simulink library "THLlib"  (R2017a)
settings: Solver=ode45  StartTime=0.0  StopTime=10.0  RelTol=1e-3  EnableMultiTasking=on
PostLoadFcn:
  | setsysloc(bdroot)
StartFcn:
  | open_system('MinSegLibrary','force')
libraries: arduinolib x6
settings Model: Creator=hurstj  LastModifiedBy=student
settings DataIOCC: LimitDataPoints=on  SaveFormat=Array  SignalLoggingSaveFormat=ModelDataLogs
settings OptimizationCC: LifeSpan=inf
settings DebuggingCC: UnderspecifiedInitializationDetection=Classic  MergeDetectMultiDrivingBlocksExec=none  SolverPrmCheckMsg=warning  MultiTaskDSMMsg=warning  MultiTaskCondExecSysMsg=none  StateNameClashWarn=warning  StrictBusMsg=None  SFUnexpectedBacktrackingDiag=warning  SFNoUnconditionalDefaultTransitionDiag=warning  SFExecutionAtInitializationDiag=none
settings HardwareCC: ProdBitPerPointer=32  ProdBitPerSizeT=32  ProdBitPerPtrDiffT=32  ProdLargestAtomicFloat=None  ProdIntDivRoundTo=Undefined  ProdEndianess=Unspecified  ProdWordSize=32  ProdHWDeviceType=32-bit Generic
settings ModelReferenceCC: PropagateSignalLabelsOutOfModel=off
settings GRTTargetCC: TargetLangStandard=C89/C90 (ANSI)  GeneratePreprocessorConditionals=Disable all
settings ConfigComp: CovMetricSettings=dw  CovHtmlReporting=on  CovSaveCumulativeToWorkspaceVar=on  CovSaveSingleToWorkspaceVar=on  CovExternalEMLEnable=off

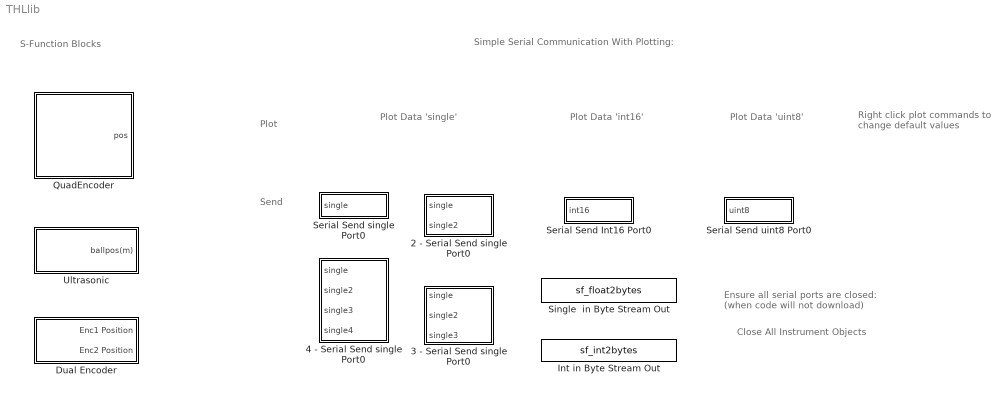
== system THLlib ==
  note: Right click
      |  plot commands
      | to change
      | default values
  note: Ensure all serial ports are closed:
      | (when code will not download)
  note: Plot
  note: Send
  note: Plot Data
      | 'int16'
  note: Plot Data
      | 'single'
  note: Plot Data
      | 'uint8'
  note: Simple Serial Communication
      | With Plotting:
  note: Close All
      | Instrument Objects
  note: S-Function Blocks
  2 - Serial Send single Port0 : Subsystem
  3 - Serial Send single Port0 : Subsystem  AncestorBlock="CSLlib/2 - Serial Send  single Port0"
  4 - Serial Send single Port0 : Subsystem  AncestorBlock="CSLlib/3 - Serial Send  single Port0"
  Dual Encoder : Subsystem
  Int in Byte Stream Out : S-Function  InitFcn=try, set_param(gcb,'FunctionName','sf_int2bytes'), end  FunctionName=sf_int2bytes  SFunctionModules=sf_int2bytes_wrapper  SFunctionDeploymentMode=off  EnableBusSupport=off  mask(S-Function Builder){}
      mask init:
      | val = [[.9  0.75 0.75 1 1 .9 .9 1]',[1 1 0.75 0.75 .9 .9 1 .9]'];try , sys = get_param(gcb,'SfunBuilderFcnName');if isempty(sys), sys = get_param(gcb,'FunctionName'); end,catch, sys = get_param(gcb,'FunctionName'); end
      settings: CopyFcn=set_param(gcb,'LinkStatus','none')  PreSaveFcn=try, set_param(gcb,'FunctionName','sf_int2bytes'), end  OpenFcn=sfunctionwizard(gcbh)
      mask Display: plot(val(:,1),val(:,2)),disp(sys), port_label('input',1,'int_in'), port_label('output',1,'bout')
  QuadEncoder : Subsystem
  Serial Send Int16 Port0 : Subsystem
  Serial Send single Port0 : Subsystem
  Serial Send uint8 Port0 : Subsystem
  Single  in Byte Stream Out : S-Function  InitFcn=try, set_param(gcb,'FunctionName','sf_float2bytes'), end  FunctionName=sf_float2bytes  SFunctionModules=sf_float2bytes_wrapper  SFunctionDeploymentMode=off  EnableBusSupport=off  mask(S-Function Builder){}
      mask init: same as THLlib/Int in Byte Stream Out
      settings: CopyFcn=set_param(gcb,'LinkStatus','none')  PreSaveFcn=try, set_param(gcb,'FunctionName','sf_float2bytes'), end  OpenFcn=sfunctionwizard(gcbh)
      mask Display: plot(val(:,1),val(:,2)),disp(sys), port_label('input',1,'fin'), port_label('output',1,'bout')
  Ultrasonic : Subsystem

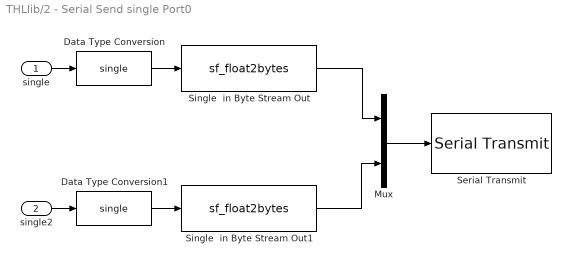
== system THLlib/2 - Serial Send single Port0 ==
  single : Inport
  single2 : Inport  Port=2
  Data Type Conversion : DataTypeConversion  OutDataTypeStr=single
  Data Type Conversion1 : DataTypeConversion  OutDataTypeStr=single
  Mux : Mux  Inputs=2
  Serial Transmit : arduinolib/Serial Transmit  portNumber=0
      settings: SourceProductName=Simulink Support Package for Arduino Hardware
  Single  in Byte Stream Out : S-Function  InitFcn=try, set_param(gcb,'FunctionName','sf_float2bytes'), end  FunctionName=sf_float2bytes  SFunctionModules=sf_float2bytes_wrapper  SFunctionDeploymentMode=off  EnableBusSupport=off  mask(S-Function Builder){}
      mask init: same as THLlib/Int in Byte Stream Out
      settings: CopyFcn=set_param(gcb,'LinkStatus','none')  PreSaveFcn=try, set_param(gcb,'FunctionName','sf_float2bytes'), end  OpenFcn=sfunctionwizard(gcbh)
      mask Display: plot(val(:,1),val(:,2)),disp(sys), port_label('input',1,'fin'), port_label('output',1,'bout')
  Single  in Byte Stream Out1 : S-Function  InitFcn=try, set_param(gcb,'FunctionName','sf_float2bytes'), end  FunctionName=sf_float2bytes  SFunctionModules=sf_float2bytes_wrapper  SFunctionDeploymentMode=off  EnableBusSupport=off  mask(S-Function Builder){}
      mask init: same as THLlib/Int in Byte Stream Out
      settings: CopyFcn=set_param(gcb,'LinkStatus','none')  PreSaveFcn=try, set_param(gcb,'FunctionName','sf_float2bytes'), end  OpenFcn=sfunctionwizard(gcbh)
      mask Display: plot(val(:,1),val(:,2)),disp(sys), port_label('input',1,'fin'), port_label('output',1,'bout')
  wires:
  Mux/1 -> Serial Transmit/1
  Single  in Byte Stream Out/1 -> Mux/1
  Single  in Byte Stream Out1/1 -> Mux/2
  Data Type Conversion1/1 -> Single  in Byte Stream Out1/1
  single2/1 -> Data Type Conversion1/1
  Data Type Conversion/1 -> Single  in Byte Stream Out/1
  single/1 -> Data Type Conversion/1

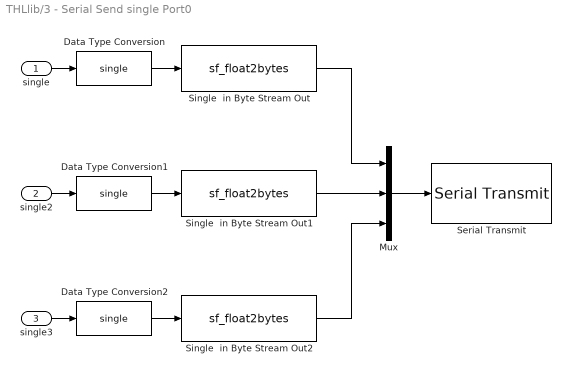
== system THLlib/3 - Serial Send single Port0 ==
  single : Inport
  single2 : Inport  Port=2
  single3 : Inport  Port=3
  Data Type Conversion : DataTypeConversion  OutDataTypeStr=single
  Data Type Conversion1 : DataTypeConversion  OutDataTypeStr=single
  Data Type Conversion2 : DataTypeConversion  OutDataTypeStr=single
  Mux : Mux  Inputs=3
  Serial Transmit : arduinolib/Serial Transmit  portNumber=0
      settings: SourceProductName=Simulink Support Package for Arduino Hardware
  Single  in Byte Stream Out : S-Function  InitFcn=try, set_param(gcb,'FunctionName','sf_float2bytes'), end  FunctionName=sf_float2bytes  SFunctionModules=sf_float2bytes_wrapper  SFunctionDeploymentMode=off  EnableBusSupport=off  mask(S-Function Builder){}
      mask init: same as THLlib/Int in Byte Stream Out
      settings: CopyFcn=set_param(gcb,'LinkStatus','none')  PreSaveFcn=try, set_param(gcb,'FunctionName','sf_float2bytes'), end  OpenFcn=sfunctionwizard(gcbh)
      mask Display: plot(val(:,1),val(:,2)),disp(sys), port_label('input',1,'fin'), port_label('output',1,'bout')
  Single  in Byte Stream Out1 : S-Function  InitFcn=try, set_param(gcb,'FunctionName','sf_float2bytes'), end  FunctionName=sf_float2bytes  SFunctionModules=sf_float2bytes_wrapper  SFunctionDeploymentMode=off  EnableBusSupport=off  mask(S-Function Builder){}
      mask init: same as THLlib/Int in Byte Stream Out
      settings: CopyFcn=set_param(gcb,'LinkStatus','none')  PreSaveFcn=try, set_param(gcb,'FunctionName','sf_float2bytes'), end  OpenFcn=sfunctionwizard(gcbh)
      mask Display: plot(val(:,1),val(:,2)),disp(sys), port_label('input',1,'fin'), port_label('output',1,'bout')
  Single  in Byte Stream Out2 : S-Function  InitFcn=try, set_param(gcb,'FunctionName','sf_float2bytes'), end  FunctionName=sf_float2bytes  SFunctionModules=sf_float2bytes_wrapper  SFunctionDeploymentMode=off  EnableBusSupport=off  mask(S-Function Builder){}
      mask init: same as THLlib/Int in Byte Stream Out
      settings: CopyFcn=set_param(gcb,'LinkStatus','none')  PreSaveFcn=try, set_param(gcb,'FunctionName','sf_float2bytes'), end  OpenFcn=sfunctionwizard(gcbh)
      mask Display: plot(val(:,1),val(:,2)),disp(sys), port_label('input',1,'fin'), port_label('output',1,'bout')
  wires:
  single/1 -> Data Type Conversion/1
  Data Type Conversion/1 -> Single  in Byte Stream Out/1
  single2/1 -> Data Type Conversion1/1
  Data Type Conversion1/1 -> Single  in Byte Stream Out1/1
  Single  in Byte Stream Out1/1 -> Mux/2
  Single  in Byte Stream Out/1 -> Mux/1
  Mux/1 -> Serial Transmit/1
  single3/1 -> Data Type Conversion2/1
  Data Type Conversion2/1 -> Single  in Byte Stream Out2/1
  Single  in Byte Stream Out2/1 -> Mux/3

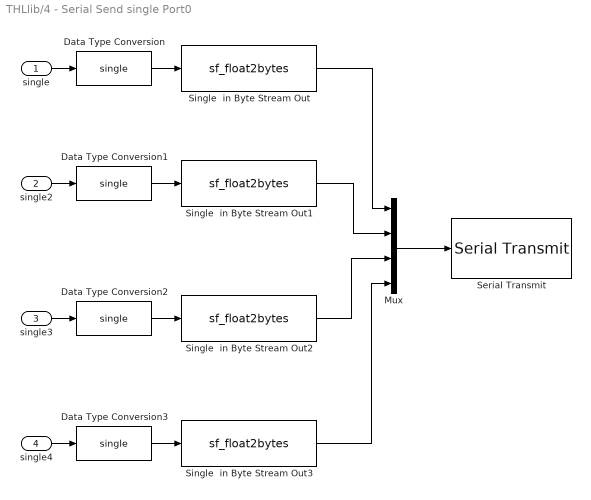
== system THLlib/4 - Serial Send single Port0 ==
  single : Inport
  single2 : Inport  Port=2
  single3 : Inport  Port=3
  single4 : Inport  Port=4
  Data Type Conversion{,1..3} (4 alike) : DataTypeConversion  OutDataTypeStr=single
  Mux : Mux
  Serial Transmit : arduinolib/Serial Transmit  portNumber=0
      settings: SourceProductName=Simulink Support Package for Arduino Hardware
  Single  in Byte Stream Out : S-Function  InitFcn=try, set_param(gcb,'FunctionName','sf_float2bytes'), end  FunctionName=sf_float2bytes  SFunctionModules=sf_float2bytes_wrapper  SFunctionDeploymentMode=off  EnableBusSupport=off  mask(S-Function Builder){}
      mask init: same as THLlib/Int in Byte Stream Out
      settings: CopyFcn=set_param(gcb,'LinkStatus','none')  PreSaveFcn=try, set_param(gcb,'FunctionName','sf_float2bytes'), end  OpenFcn=sfunctionwizard(gcbh)
      mask Display: plot(val(:,1),val(:,2)),disp(sys), port_label('input',1,'fin'), port_label('output',1,'bout')
  Single  in Byte Stream Out1 : S-Function  InitFcn=try, set_param(gcb,'FunctionName','sf_float2bytes'), end  FunctionName=sf_float2bytes  SFunctionModules=sf_float2bytes_wrapper  SFunctionDeploymentMode=off  EnableBusSupport=off  mask(S-Function Builder){}
      mask init: same as THLlib/Int in Byte Stream Out
      settings: CopyFcn=set_param(gcb,'LinkStatus','none')  PreSaveFcn=try, set_param(gcb,'FunctionName','sf_float2bytes'), end  OpenFcn=sfunctionwizard(gcbh)
      mask Display: plot(val(:,1),val(:,2)),disp(sys), port_label('input',1,'fin'), port_label('output',1,'bout')
  Single  in Byte Stream Out2 : S-Function  InitFcn=try, set_param(gcb,'FunctionName','sf_float2bytes'), end  FunctionName=sf_float2bytes  SFunctionModules=sf_float2bytes_wrapper  SFunctionDeploymentMode=off  EnableBusSupport=off  mask(S-Function Builder){}
      mask init: same as THLlib/Int in Byte Stream Out
      settings: CopyFcn=set_param(gcb,'LinkStatus','none')  PreSaveFcn=try, set_param(gcb,'FunctionName','sf_float2bytes'), end  OpenFcn=sfunctionwizard(gcbh)
      mask Display: plot(val(:,1),val(:,2)),disp(sys), port_label('input',1,'fin'), port_label('output',1,'bout')
  Single  in Byte Stream Out3 : S-Function  InitFcn=try, set_param(gcb,'FunctionName','sf_float2bytes'), end  FunctionName=sf_float2bytes  SFunctionModules=sf_float2bytes_wrapper  SFunctionDeploymentMode=off  EnableBusSupport=off  mask(S-Function Builder){}
      mask init: same as THLlib/Int in Byte Stream Out
      settings: CopyFcn=set_param(gcb,'LinkStatus','none')  PreSaveFcn=try, set_param(gcb,'FunctionName','sf_float2bytes'), end  OpenFcn=sfunctionwizard(gcbh)
      mask Display: plot(val(:,1),val(:,2)),disp(sys), port_label('input',1,'fin'), port_label('output',1,'bout')
  wires:
  Single  in Byte Stream Out2/1 -> Mux/3
  Data Type Conversion2/1 -> Single  in Byte Stream Out2/1
  single3/1 -> Data Type Conversion2/1
  Mux/1 -> Serial Transmit/1
  Single  in Byte Stream Out/1 -> Mux/1
  Single  in Byte Stream Out1/1 -> Mux/2
  Data Type Conversion1/1 -> Single  in Byte Stream Out1/1
  single2/1 -> Data Type Conversion1/1
  Data Type Conversion/1 -> Single  in Byte Stream Out/1
  single/1 -> Data Type Conversion/1
  Data Type Conversion3/1 -> Single  in Byte Stream Out3/1
  single4/1 -> Data Type Conversion3/1
  Single  in Byte Stream Out3/1 -> Mux/4

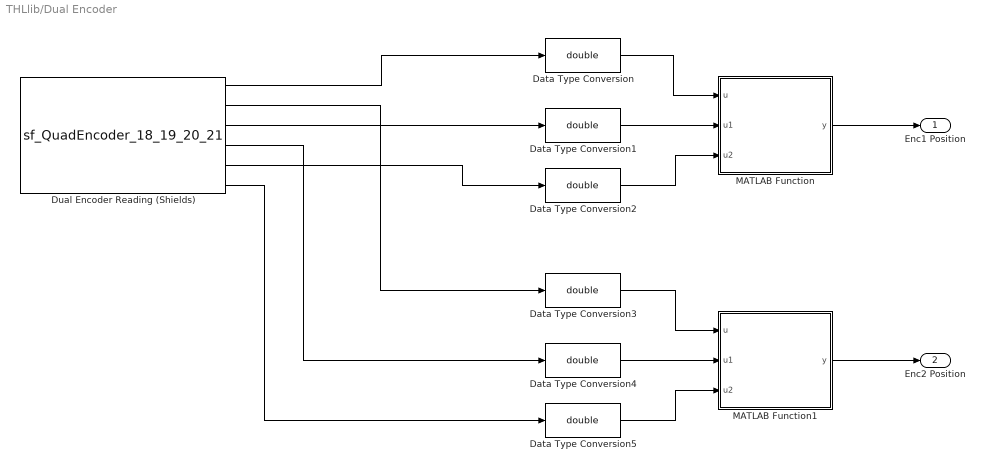
== system THLlib/Dual Encoder ==
  Data Type Conversion{,1..5} (6 alike) : DataTypeConversion  OutDataTypeStr=double
  Dual Encoder Reading (Shields) : S-Function  InitFcn=try, set_param(gcb,'FunctionName','sf_QuadEncoder_18_19_20_21'), end  FunctionName=sf_QuadEncoder_18_19_20_21  Parameters=uint8([0 1]),uint8([18 20]),uint8([19 21])  SFunctionModules=sf_QuadEncoder_18_19_20_21_wrapper  SFunctionDeploymentMode=off  EnableBusSupport=off  mask(S-Function Builder){}
      mask init: same as THLlib/Int in Byte Stream Out
      settings: CopyFcn=set_param(gcbh,'LinkStatus','none')  PreSaveFcn=try, set_param(gcb,'FunctionName','sf_QuadEncoder_18_19_20_21'), end  OpenFcn=sfunctionwizard(gcbh)
      mask Display: plot(val(:,1),val(:,2)),disp(sys), port_label('output',1,'pos1'), port_label('output',2,'pos2'), port_label('output',3,'OF1'), port_label('output',4,'OF2'), port_label('output',5,'UF1'), port_label('output',6,'UF2')
  MATLAB Function : Subsystem  TreatAsAtomicUnit=on
  MATLAB Function1 : Subsystem  TreatAsAtomicUnit=on
  Enc1 Position : Outport
  Enc2 Position : Outport  Port=2
  wires:
  MATLAB Function1/1(y) -> Enc2 Position/1
  MATLAB Function/1(y) -> Enc1 Position/1
  Data Type Conversion5/1 -> MATLAB Function1/3(u2)
  Data Type Conversion4/1 -> MATLAB Function1/2(u1)
  Data Type Conversion3/1 -> MATLAB Function1/1(u)
  Data Type Conversion2/1 -> MATLAB Function/3(u2)
  Data Type Conversion1/1 -> MATLAB Function/2(u1)
  Data Type Conversion/1 -> MATLAB Function/1(u)
  Dual Encoder Reading (Shields)/6 -> Data Type Conversion5/1
  Dual Encoder Reading (Shields)/5 -> Data Type Conversion2/1
  Dual Encoder Reading (Shields)/4 -> Data Type Conversion4/1
  Dual Encoder Reading (Shields)/3 -> Data Type Conversion1/1
  Dual Encoder Reading (Shields)/2 -> Data Type Conversion3/1
  Dual Encoder Reading (Shields)/1 -> Data Type Conversion/1

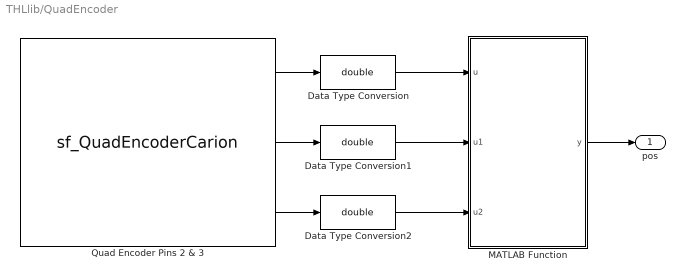
== system THLlib/QuadEncoder ==
  Data Type Conversion : DataTypeConversion  OutDataTypeStr=double
  Data Type Conversion1 : DataTypeConversion  OutDataTypeStr=double
  Data Type Conversion2 : DataTypeConversion  OutDataTypeStr=double
  MATLAB Function : MATLAB Function  TreatAsAtomicUnit=on
  Quad Encoder Pins 2 & 3 : S-Function  InitFcn=try, set_param(gcb,'FunctionName','sf_QuadEncoderCarion'), end  FunctionName=sf_QuadEncoderCarion  Parameters=uint8(0),uint8(2),uint8(3)  SFunctionModules=sf_QuadEncoderCarion_wrapper  SFunctionDeploymentMode=off  EnableBusSupport=off  mask(S-Function Builder){}
      mask init: same as THLlib/Int in Byte Stream Out
      settings: CopyFcn=set_param(gcbh,'LinkStatus','none')  PreSaveFcn=try, set_param(gcb,'FunctionName','sf_QuadEncoderCarion'), end  OpenFcn=sfunctionwizard(gcbh)
      mask Display: plot(val(:,1),val(:,2)),disp(sys), port_label('output',1,'pos'), port_label('output',2,'overflow'), port_label('output',3,'underflow')
  pos : Outport
  wires:
  Quad Encoder Pins 2 & 3/3 -> Data Type Conversion2/1
  Quad Encoder Pins 2 & 3/2 -> Data Type Conversion1/1
  MATLAB Function/1(y) -> pos/1
  Quad Encoder Pins 2 & 3/1 -> Data Type Conversion/1
  Data Type Conversion2/1 -> MATLAB Function/3(u2)
  Data Type Conversion1/1 -> MATLAB Function/2(u1)
  Data Type Conversion/1 -> MATLAB Function/1(u)

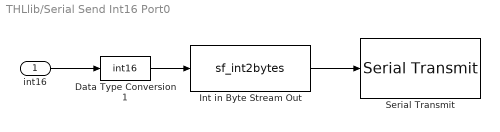
== system THLlib/Serial Send Int16 Port0 ==
  int16 : Inport
  Data Type Conversion1 : DataTypeConversion  OutDataTypeStr=int16
  Int in Byte Stream Out : S-Function  InitFcn=try, set_param(gcb,'FunctionName','sf_int2bytes'), end  FunctionName=sf_int2bytes  SFunctionModules=sf_int2bytes_wrapper  SFunctionDeploymentMode=off  EnableBusSupport=off  mask(S-Function Builder){}
      mask init: same as THLlib/Int in Byte Stream Out
      settings: CopyFcn=set_param(gcb,'LinkStatus','none')  PreSaveFcn=try, set_param(gcb,'FunctionName','sf_int2bytes'), end  OpenFcn=sfunctionwizard(gcbh)
      mask Display: plot(val(:,1),val(:,2)),disp(sys), port_label('input',1,'int_in'), port_label('output',1,'bout')
  Serial Transmit : arduinolib/Serial Transmit  portNumber=0
      settings: SourceProductName=Simulink Support Package for Arduino Hardware
  wires:
  Data Type Conversion1/1 -> Int in Byte Stream Out/1
  int16/1 -> Data Type Conversion1/1
  Int in Byte Stream Out/1 -> Serial Transmit/1

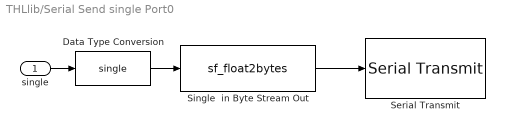
== system THLlib/Serial Send single Port0 ==
  single : Inport
  Data Type Conversion : DataTypeConversion  OutDataTypeStr=single
  Serial Transmit : arduinolib/Serial Transmit  portNumber=0
      settings: SourceProductName=Simulink Support Package for Arduino Hardware
  Single  in Byte Stream Out : S-Function  InitFcn=try, set_param(gcb,'FunctionName','sf_float2bytes'), end  FunctionName=sf_float2bytes  SFunctionModules=sf_float2bytes_wrapper  SFunctionDeploymentMode=off  EnableBusSupport=off  mask(S-Function Builder){}
      mask init: same as THLlib/Int in Byte Stream Out
      settings: CopyFcn=set_param(gcb,'LinkStatus','none')  PreSaveFcn=try, set_param(gcb,'FunctionName','sf_float2bytes'), end  OpenFcn=sfunctionwizard(gcbh)
      mask Display: plot(val(:,1),val(:,2)),disp(sys), port_label('input',1,'fin'), port_label('output',1,'bout')
  wires:
  Single  in Byte Stream Out/1 -> Serial Transmit/1
  Data Type Conversion/1 -> Single  in Byte Stream Out/1
  single/1 -> Data Type Conversion/1

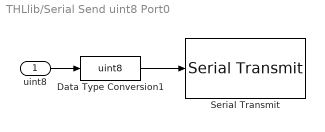
== system THLlib/Serial Send uint8 Port0 ==
  uint8 : Inport
  Data Type Conversion1 : DataTypeConversion  OutDataTypeStr=uint8
  Serial Transmit : arduinolib/Serial Transmit  portNumber=0
      settings: SourceProductName=Simulink Support Package for Arduino Hardware
  wires:
  uint8/1 -> Data Type Conversion1/1
  Data Type Conversion1/1 -> Serial Transmit/1

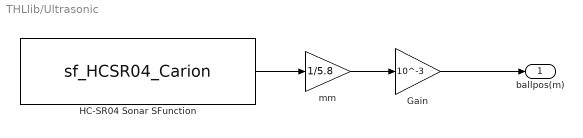
== system THLlib/Ultrasonic ==
  Gain : Gain  Gain=10^-3
  HC-SR04 Sonar SFunction : S-Function  InitFcn=try, set_param(gcb,'FunctionName','sf_HCSR04_Carion'), end  FunctionName=sf_HCSR04_Carion  SFunctionModules=sf_HCSR04_Carion_wrapper  SFunctionDeploymentMode=off  EnableBusSupport=off  mask(S-Function Builder){}
      mask help: Simulink:masks:SFunctionBuilder_MD
      mask init: same as THLlib/Int in Byte Stream Out
      settings: CopyFcn=set_param(gcbh,'LinkStatus','none')  PreSaveFcn=try, set_param(gcb,'FunctionName','sf_HCSR04_Carion'), end  OpenFcn=sfunctionwizard(gcbh)
      mask Display: plot(val(:,1),val(:,2)),disp(sys), port_label('output',1,'distance_us')
  mm : Gain  Gain=1/5.8
  ballpos(m) : Outport
  wires:
  Gain/1 -> ballpos(m)/1
  mm/1 -> Gain/1
  HC-SR04 Sonar SFunction/1 -> mm/1

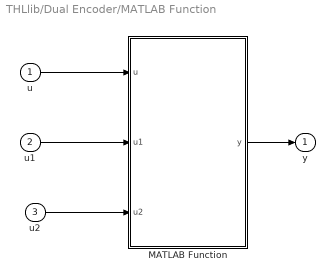
== system THLlib/Dual Encoder/MATLAB Function ==
  u : Inport
  u1 : Inport  Port=2
  u2 : Inport  Port=3
  MATLAB Function : MATLAB Function  TreatAsAtomicUnit=on
  y : Outport
  wires:
  MATLAB Function/1(y) -> y/1
  u1/1 -> MATLAB Function/2(u1)
  u2/1 -> MATLAB Function/3(u2)
  u/1 -> MATLAB Function/1(u)

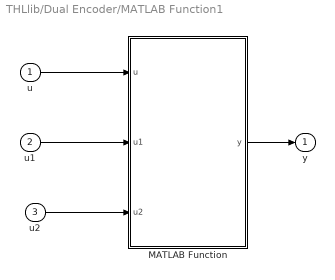
== system THLlib/Dual Encoder/MATLAB Function1 ==
  u : Inport
  u1 : Inport  Port=2
  u2 : Inport  Port=3
  MATLAB Function : MATLAB Function  TreatAsAtomicUnit=on
  y : Outport
  wires:
  MATLAB Function/1(y) -> y/1
  u1/1 -> MATLAB Function/2(u1)
  u2/1 -> MATLAB Function/3(u2)
  u/1 -> MATLAB Function/1(u)

== matlab function THLlib/QuadEncoder/MATLAB Function ==
  data: u input; y output; u1 input; u2 input
function y = fcn(u,u1,u2)
%#codegen
max = 32767;
min = -32767;

y = u1*max + u2*min + u;

== matlab function THLlib/Dual Encoder/MATLAB Function/MATLAB Function ==
  data: u input; y output; u1 input; u2 input
function y = fcn(u,u1,u2)
%#codegen
max = 32767;
min = -32767;

y = u1*max + u2*min + u;

== matlab function THLlib/Dual Encoder/MATLAB Function1/MATLAB Function ==
  data: u input; y output; u1 input; u2 input
function y = fcn(u,u1,u2)
%#codegen
max = 32767;
min = -32767;

y = u1*max + u2*min + u;
